simulink model "low_pass_filter"  (R2013a)
settings: Solver=ode45  StartTime=0.0  StopTime=10.0  RelTol=1e-3
values from neighbouring files (symbols this model uses):
  dcAd = dcinvexp*(eye(dcnstates) + (Ts/2)*dcAc)    [charging_lpf.m]    (also in lpf_params.m; protection_lpf.m)
  dcBd = dcinvexp*dcBc    [charging_lpf.m]    (also in lpf_params.m; protection_lpf.m)
  dcCd = dcCc*dcinvexp*Ts    [charging_lpf.m]    (also in lpf_params.m; protection_lpf.m)
  dcDd = dcCc*dcinvexp*dcBc*(Ts/2) + dcDc    [charging_lpf.m]    (also in lpf_params.m; protection_lpf.m)
  Ts = 1/20000    (= 5e-05)    [charging_lpf.m]    (also in lpf_params.m = 0.001; protection_lpf.m)
settings Model: Creator=50c  LastModifiedBy=50c

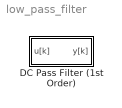
== system low_pass_filter ==
  DC Pass Filter (1st Order) : Subsystem  mask{dc_filter_Ts=5e-5}
      mask prompts: dc_filter_Ts "Sample Time"
      mask help: Low Pass Filter to provide unity gain and 0 phase shift at DC

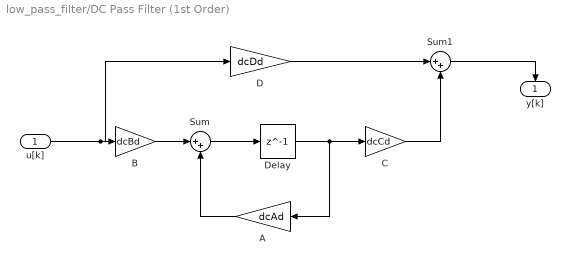
== system low_pass_filter/DC Pass Filter (1st Order) ==
  u[k] : Inport
  A : Gain  Gain=dcAd
  B : Gain  Gain=dcBd
  C : Gain  Gain=dcCd
  D : Gain  Gain=dcDd
  Delay : Delay  DelayLength=1  InitialCondition=0  SampleTime=Ts
  Sum : Sum  Inputs=|++
  Sum1 : Sum  Inputs=|++
  y[k] : Outport
  wires:
  B/1 -> Sum/1
  u[k]/1 -> D/1, B/1
  Sum1/1 -> y[k]/1
  Delay/1 -> A/1, C/1
  Sum/1 -> Delay/1
  D/1 -> Sum1/1
  A/1 -> Sum/2
  C/1 -> Sum1/2
